simulink library "motion"  (Simulink 4.00)
undefined symbols (not defined in the file or in its folder): A6, Ac, Acd, ad, Aff, Aff0, Aff6, Ap, As, B6, Bc, Bcd, Bff, Bff0, Bff6, Bp, Bs, C6, Cc, Ccd, Cff, Cff0, Cff6, Cp, Cs, D6, Dc, dd, Ddd, Dff, Dff0, Dff6, Dp, Ds, jd, Ts, Tsettle
libraries: motion x5
(part 3 of 4)

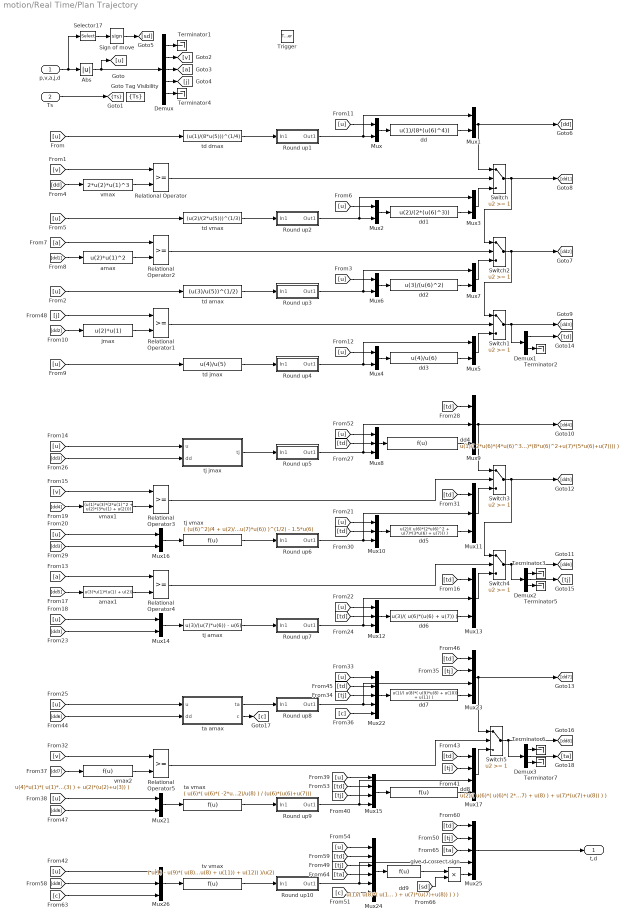
== system motion/Real Time/Plan Trajectory ==
  p,v,a,j,d : Inport  Port=1
  Ts : Inport  Port=2
  Trigger : TriggerPort  TriggerType=rising  OutputDataType=auto
  Abs : Abs  SaturateOnIntegerOverflow=on
  Demux : Demux  Outputs=5  BusSelectionMode=off
  Demux1 : Demux  Outputs=2  BusSelectionMode=off
  Demux2 : Demux  Outputs=3  BusSelectionMode=off
  Demux3 : Demux  Outputs=[2 1 1]  BusSelectionMode=off
  Goto Tag Visibility : GotoTagVisibility  GotoTag=Ts
  Mux{,1..7,14,16,21} (11 alike) : Mux  Inputs=2
  Mux{8..13,26} (7 alike) : Mux  Inputs=3
  Mux15 : Mux  Inputs=4
  Mux17 : Mux  Inputs=4
  Mux22 : Mux  Inputs=5
  Mux23 : Mux  Inputs=4
  Mux24 : Mux  Inputs=6
  Mux25 : Mux  Inputs=5
  Relational Operator{,1..5} (6 alike) : RelationalOperator  Operator=>=
  Round up1 : Subsystem
      settings: RTWFcnNameOpts=Auto  RTWFileNameOpts=Auto
      mask Display: disp('Ts*ceil(u/Ts)')
  Round up10 : Subsystem
      settings: RTWFcnNameOpts=Auto  RTWFileNameOpts=Auto
      mask Display: disp('Ts*ceil(u/Ts)')
  Round up2 : Subsystem
      settings: RTWFcnNameOpts=Auto  RTWFileNameOpts=Auto
      mask Display: disp('Ts*ceil(u/Ts)')
  Round up3 : Subsystem
      settings: RTWFcnNameOpts=Auto  RTWFileNameOpts=Auto
      mask Display: disp('Ts*ceil(u/Ts)')
  Round up4 : Subsystem
      settings: RTWFcnNameOpts=Auto  RTWFileNameOpts=Auto
      mask Display: disp('Ts*ceil(u/Ts)')
  Round up5 : Subsystem
      settings: RTWFcnNameOpts=Auto  RTWFileNameOpts=Auto
      mask Display: disp('Ts*ceil(u/Ts)')
  Round up6 : Subsystem
      settings: RTWFcnNameOpts=Auto  RTWFileNameOpts=Auto
      mask Display: disp('Ts*ceil(u/Ts)')
  Round up7 : Subsystem
      settings: RTWFcnNameOpts=Auto  RTWFileNameOpts=Auto
      mask Display: disp('Ts*ceil(u/Ts)')
  Round up8 : Subsystem
      settings: RTWFcnNameOpts=Auto  RTWFileNameOpts=Auto
      mask Display: disp('Ts*ceil(u/Ts)')
  Round up9 : Subsystem
      settings: RTWFcnNameOpts=Auto  RTWFileNameOpts=Auto
      mask Display: disp('Ts*ceil(u/Ts)')
  Selector17 : Selector  InputType=Vector  ElementSrc=Internal  Elements=1  RowSrc=Internal  Rows=1  ColumnSrc=Internal  Columns=1  InputPortWidth=5
  Sign of move : Signum
  Switch{,1..5} (6 alike) : Switch  Threshold=1
  Terminator{1..7} (7 alike) : Terminator
  amax : Fcn  Expr=u(2)*u(1)^2
  amax1 : Fcn  Expr=u(3)*u(1)*(u(1) + u(2))
  dd : Fcn  Expr=u(1)/(8*(u(6)^4))
  dd1 : Fcn  Expr=u(2)/(2*(u(6)^3))
  dd2 : Fcn  Expr=u(3)/(u(6)^2)
  dd3 : Fcn  Expr=u(4)/u(6)
  dd4 : Fcn  Expr=u(1)/( 2*u(6)*(4*u(6)^3+u(7)*(8*u(6)^2+u(7)*(5*u(6)+u(7)))) )
  dd5 : Fcn  Expr=u(2)/( u(6)*(2*u(6)^2 + u(7)*(3*u(6) + u(7))) )
  dd6 : Fcn  Expr=u(3)/( u(6)*(u(6) + u(7)) )
  dd7 : Fcn  Expr=u(1)/( u(8)*( u(9)*u(8) + u(10)) + u(11) )
  dd8 : Fcn  Expr=u(2)/( u(6)*( u(6)*( 2*u(6) + 3*u(7) + u(8) ) + u(7)*(u(7)+u(8)) ) )
  dd9 : Fcn  Expr=u(1)/( u(8)*( u(10)*u(8) + u(11)) + u(12) + u(9)*( u(6)*( u(6)*( 2*u(6) + 3*u(7) + u(8) ) + u(7)*(u(7)+u(8)) ) ) )
  give d correct sign : Product  Inputs=2  Multiplication=Element-wise(.*)  SaturateOnIntegerOverflow=on
  jmax : Fcn  Expr=u(2)*u(1)
  ta amax : Subsystem
      settings: RTWFcnNameOpts=Auto  RTWFileNameOpts=Auto
  ta vmax : Fcn  Expr=( u(6)*( u(6)*( -2*u(6) - 3*u(7) ) - u(7)^2 ) + u(2)/u(8) ) / (u(6)*(u(6)+u(7)))
  td amax : Fcn  Expr=(u(3)/u(5))^(1/2)
  td dmax : Fcn  Expr=(u(1)/(8*u(5)))^(1/4)
  td jmax : Fcn  Expr=u(4)/u(5)
  td vmax : Fcn  Expr=(u(2)/(2*u(5)))^(1/3)
  tj amax : Fcn  Expr=u(3)/(u(7)*u(6)) - u(6)
  tj jmax : Subsystem
      settings: RTWFcnNameOpts=Auto  RTWFileNameOpts=Auto
  tj vmax : Fcn  Expr=( (u(6)^2)/4 + u(2)/(u(7)*u(6)) )^(1/2) - 1.5*u(6)
  tv vmax : Fcn  Expr=( u(1) - u(9)*( u(8)*(u(10)*u(8) + u(11)) + u(12)) )/u(2)
  vmax : Fcn  Expr=2*u(2)*u(1)^3
  vmax1 : Fcn  Expr=(u(1)*u(3)*(2*u(1)^2 + u(2)*(3*u(1) + u(2))))
  vmax2 : Fcn  Expr=u(4)*u(1)*( u(1)*( 2*u(1) + 3*u(2) + u(3) ) + u(2)*(u(2)+u(3)) )
  t,d : Outport  Port=1
  tag scope: Ts=scoped
  wires:
  [sd] -> give d correct sign/2
  dd9/1 -> give d correct sign/1
  give d correct sign/1 -> Mux25/5
  [ta] -> Mux25/3
  [tj] -> Mux25/2
  [td] -> Mux25/1
  Mux25/1 -> t,d/1
  Sign of move/1 -> [sd]
  Selector17/1 -> Sign of move/1
  p,v,a,j,d/1 -> Selector17/1, Abs/1
  Abs/1 -> Demux/1, [u]
  Demux/5 -> Terminator4/1
  Demux/4 -> [j]
  Demux/3 -> [a]
  Demux/2 -> [v]
  Demux/1 -> Terminator1/1
  Ts/1 -> [Ts]
  Round up10/1(Out1) -> Mux24/5, Mux25/4
  tv vmax/1 -> Round up10/1(In1)
  Round up9/1(Out1) -> Mux15/4, Mux17/3
  ta vmax/1 -> Round up9/1(In1)
  Round up8/1(Out1) -> Mux22/4, Mux23/3
  ta amax/1(ta) -> Round up8/1(In1)
  Round up7/1(Out1) -> Mux12/3, Mux13/2
  tj amax/1 -> Round up7/1(In1)
  Round up6/1(Out1) -> Mux10/3, Mux11/2
  tj vmax/1 -> Round up6/1(In1)
  Round up5/1(Out1) -> Mux8/3, Mux9/2
  tj jmax/1(tj) -> Round up5/1(In1)
  Round up4/1(Out1) -> Mux4/2, Mux5/1
  td jmax/1 -> Round up4/1(In1)
  Round up3/1(Out1) -> Mux7/1, Mux6/2
  td amax/1 -> Round up3/1(In1)
  Round up2/1(Out1) -> Mux2/2, Mux3/1
  vmax2/1 -> Relational Operator5/2
  [v] -> Relational Operator5/1
  amax1/1 -> Relational Operator4/2
  [a] -> Relational Operator4/1
  vmax1/1 -> Relational Operator3/2
  [v] -> Relational Operator3/1
  [u] -> Mux24/1
  [u] -> Mux26/1
  Demux3/3 -> Terminator7/1
  Demux3/1 -> Terminator6/1
  Demux3/2 -> [ta]
  Switch5/1 -> Demux3/1, [dd8]
  Relational Operator5/1 -> Switch5/2
  Mux17/1 -> Switch5/3
  [u] -> Mux22/1
  [tj] -> Mux17/2
  [td] -> Mux17/1
  [tj] -> Mux15/3
  ta amax/2(c) -> [c]
  [c] -> Mux22/5
  [tj] -> Mux23/2
  [tj] -> Mux22/3
  [td] -> Mux15/2
  [dd6] -> Mux21/2
  Mux21/1 -> ta vmax/1
  [u] -> Mux21/1
  [td] -> Mux23/1
  [td] -> Mux22/2
  [dd6] -> ta amax/2(dd)
  Mux15/1 -> dd8/1
  dd8/1 -> Mux17/4
  [u] -> Mux15/1
  Mux23/1 -> Switch5/1, [dd7]
  [dd7] -> vmax2/1
  dd7/1 -> Mux23/4
  Mux22/1 -> dd7/1
  [u] -> ta amax/1(u)
  Demux2/3 -> Terminator5/1
  Demux2/1 -> Terminator3/1
  Demux2/2 -> [tj]
  Switch4/1 -> Demux2/1, [dd6]
  Relational Operator4/1 -> Switch4/2
  Mux13/1 -> Switch4/3
  Switch3/1 -> Switch4/1, [dd5]
  Relational Operator3/1 -> Switch3/2
  Mux11/1 -> Switch3/3
  [u] -> Mux8/1
  [td] -> Mux13/1
  [td] -> Mux12/2
  [dd3] -> Mux14/2
  Mux14/1 -> tj amax/1
  [u] -> Mux14/1
  Mux12/1 -> dd6/1
  dd6/1 -> Mux13/3
  [u] -> Mux12/1
  [dd5] -> amax1/1
  [td] -> Mux11/1
  [td] -> Mux10/2
  [dd3] -> Mux16/2
  Mux16/1 -> tj vmax/1
  [u] -> Mux16/1
  [td] -> Mux9/1
  [td] -> Mux8/2
  [dd3] -> tj jmax/2(dd)
  Mux10/1 -> dd5/1
  dd5/1 -> Mux11/3
  [u] -> Mux10/1
  Mux9/1 -> Switch3/1, [dd4]
  [dd4] -> vmax1/1
  dd4/1 -> Mux9/3
  Mux8/1 -> dd4/1
  [u] -> tj jmax/1(u)
  Demux1/2 -> Terminator2/1
  Demux1/1 -> [td]
  [u] -> Mux/1
  jmax/1 -> Relational Operator1/2
  [j] -> Relational Operator1/1
  Switch1/1 -> Demux1/1, [dd3]
  Relational Operator1/1 -> Switch1/2
  Mux5/1 -> Switch1/3
  Mux4/1 -> dd3/1
  dd3/1 -> Mux5/2
  [u] -> Mux4/1
  [u] -> td jmax/1
  [dd2] -> jmax/1
  amax/1 -> Relational Operator2/2
  [a] -> Relational Operator2/1
  Switch2/1 -> Switch1/1, [dd2]
  Relational Operator2/1 -> Switch2/2
  Mux7/1 -> Switch2/3
  Mux6/1 -> dd2/1
  dd2/1 -> Mux7/2
  [u] -> Mux6/1
  [u] -> td amax/1
  [dd1] -> amax/1
  vmax/1 -> Relational Operator/2
  [v] -> Relational Operator/1
  Switch/1 -> Switch2/1, [dd1]
  Relational Operator/1 -> Switch/2
  Mux3/1 -> Switch/3
  td vmax/1 -> Round up2/1(In1)
  Mux2/1 -> dd1/1
  dd1/1 -> Mux3/2
  [u] -> Mux2/1
  [u] -> td vmax/1
  Mux1/1 -> Switch/1, [dd]
  [dd] -> vmax/1
  dd/1 -> Mux1/2
  Mux/1 -> dd/1
  Round up1/1(Out1) -> Mux/2, Mux1/1
  td dmax/1 -> Round up1/1(In1)
  [u] -> td dmax/1
  [ta] -> Mux24/4
  [c] -> Mux24/6
  [c] -> Mux26/3
  Mux26/1 -> tv vmax/1
  [tj] -> Mux24/3
  [td] -> Mux24/2
  [dd8] -> Mux26/2
  Mux24/1 -> dd9/1

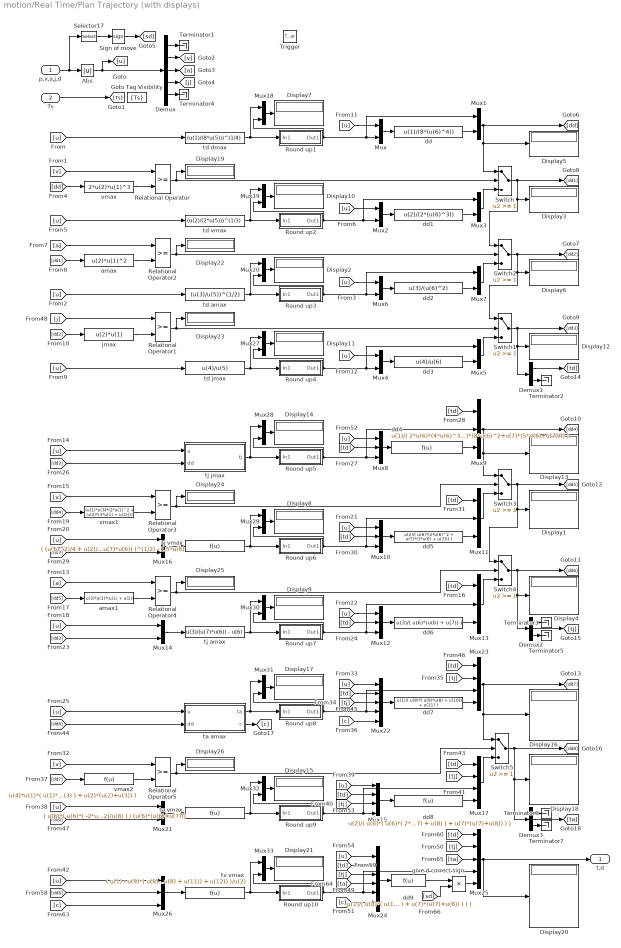
== system motion/Real Time/Plan Trajectory (with displays) ==
  p,v,a,j,d : Inport  Port=1
  Ts : Inport  Port=2
  Trigger : TriggerPort  TriggerType=rising  OutputDataType=auto
  Abs : Abs  SaturateOnIntegerOverflow=on
  Demux : Demux  Outputs=5  BusSelectionMode=off
  Demux1 : Demux  Outputs=2  BusSelectionMode=off
  Demux2 : Demux  Outputs=3  BusSelectionMode=off
  Demux3 : Demux  Outputs=[2 1 1]  BusSelectionMode=off
  Display{1..26} (26 alike) : Display
      settings: Format=short
  Goto Tag Visibility : GotoTagVisibility  GotoTag=Ts
  Mux{,1..7,14,16,18..21,27..33} (21 alike) : Mux  Inputs=2
  Mux{8..13,26} (7 alike) : Mux  Inputs=3
  Mux15 : Mux  Inputs=4
  Mux17 : Mux  Inputs=4
  Mux22 : Mux  Inputs=5
  Mux23 : Mux  Inputs=4
  Mux24 : Mux  Inputs=6
  Mux25 : Mux  Inputs=5
  Relational Operator{,1..5} (6 alike) : RelationalOperator  Operator=>=
  Round up1 : Subsystem
      settings: RTWFcnNameOpts=Auto  RTWFileNameOpts=Auto
      mask Display: disp('Ts*ceil(u/Ts)')
  Round up10 : Subsystem
      settings: RTWFcnNameOpts=Auto  RTWFileNameOpts=Auto
      mask Display: disp('Ts*ceil(u/Ts)')
  Round up2 : Subsystem
      settings: RTWFcnNameOpts=Auto  RTWFileNameOpts=Auto
      mask Display: disp('Ts*ceil(u/Ts)')
  Round up3 : Subsystem
      settings: RTWFcnNameOpts=Auto  RTWFileNameOpts=Auto
      mask Display: disp('Ts*ceil(u/Ts)')
  Round up4 : Subsystem
      settings: RTWFcnNameOpts=Auto  RTWFileNameOpts=Auto
      mask Display: disp('Ts*ceil(u/Ts)')
  Round up5 : Subsystem
      settings: RTWFcnNameOpts=Auto  RTWFileNameOpts=Auto
      mask Display: disp('Ts*ceil(u/Ts)')
  Round up6 : Subsystem
      settings: RTWFcnNameOpts=Auto  RTWFileNameOpts=Auto
      mask Display: disp('Ts*ceil(u/Ts)')
  Round up7 : Subsystem
      settings: RTWFcnNameOpts=Auto  RTWFileNameOpts=Auto
      mask Display: disp('Ts*ceil(u/Ts)')
  Round up8 : Subsystem
      settings: RTWFcnNameOpts=Auto  RTWFileNameOpts=Auto
      mask Display: disp('Ts*ceil(u/Ts)')
  Round up9 : Subsystem
      settings: RTWFcnNameOpts=Auto  RTWFileNameOpts=Auto
      mask Display: disp('Ts*ceil(u/Ts)')
  Selector17 : Selector  InputType=Vector  ElementSrc=Internal  Elements=1  RowSrc=Internal  Rows=1  ColumnSrc=Internal  Columns=1  InputPortWidth=5
  Sign of move : Signum
  Switch{,1..5} (6 alike) : Switch  Threshold=1
  Terminator{1..7} (7 alike) : Terminator
  amax : Fcn  Expr=u(2)*u(1)^2
  amax1 : Fcn  Expr=u(3)*u(1)*(u(1) + u(2))
  dd : Fcn  Expr=u(1)/(8*(u(6)^4))
  dd1 : Fcn  Expr=u(2)/(2*(u(6)^3))
  dd2 : Fcn  Expr=u(3)/(u(6)^2)
  dd3 : Fcn  Expr=u(4)/u(6)
  dd4 : Fcn  Expr=u(1)/( 2*u(6)*(4*u(6)^3+u(7)*(8*u(6)^2+u(7)*(5*u(6)+u(7)))) )
  dd5 : Fcn  Expr=u(2)/( u(6)*(2*u(6)^2 + u(7)*(3*u(6) + u(7))) )
  dd6 : Fcn  Expr=u(3)/( u(6)*(u(6) + u(7)) )
  dd7 : Fcn  Expr=u(1)/( u(8)*( u(9)*u(8) + u(10)) + u(11) )
  dd8 : Fcn  Expr=u(2)/( u(6)*( u(6)*( 2*u(6) + 3*u(7) + u(8) ) + u(7)*(u(7)+u(8)) ) )
  dd9 : Fcn  Expr=u(1)/( u(8)*( u(10)*u(8) + u(11)) + u(12) + u(9)*( u(6)*( u(6)*( 2*u(6) + 3*u(7) + u(8) ) + u(7)*(u(7)+u(8)) ) ) )
  give d correct sign : Product  Inputs=2  Multiplication=Element-wise(.*)  SaturateOnIntegerOverflow=on
  jmax : Fcn  Expr=u(2)*u(1)
  ta amax : Subsystem
      settings: RTWFcnNameOpts=Auto  RTWFileNameOpts=Auto
  ta vmax : Fcn  Expr=( u(6)*( u(6)*( -2*u(6) - 3*u(7) ) - u(7)^2 ) + u(2)/u(8) ) / (u(6)*(u(6)+u(7)))
  td amax : Fcn  Expr=(u(3)/u(5))^(1/2)
  td dmax : Fcn  Expr=(u(1)/(8*u(5)))^(1/4)
  td jmax : Fcn  Expr=u(4)/u(5)
  td vmax : Fcn  Expr=(u(2)/(2*u(5)))^(1/3)
  tj amax : Fcn  Expr=u(3)/(u(7)*u(6)) - u(6)
  tj jmax : Subsystem
      settings: RTWFcnNameOpts=Auto  RTWFileNameOpts=Auto
  tj vmax : Fcn  Expr=( (u(6)^2)/4 + u(2)/(u(7)*u(6)) )^(1/2) - 1.5*u(6)
  tv vmax : Fcn  Expr=( u(1) - u(9)*( u(8)*(u(10)*u(8) + u(11)) + u(12)) )/u(2)
  vmax : Fcn  Expr=2*u(2)*u(1)^3
  vmax1 : Fcn  Expr=(u(1)*u(3)*(2*u(1)^2 + u(2)*(3*u(1) + u(2))))
  vmax2 : Fcn  Expr=u(4)*u(1)*( u(1)*( 2*u(1) + 3*u(2) + u(3) ) + u(2)*(u(2)+u(3)) )
  t,d : Outport  Port=1
  tag scope: Ts=scoped
  wires:
  Mux24/1 -> dd9/1
  [dd8] -> Mux26/2
  [td] -> Mux24/2
  [tj] -> Mux24/3
  Mux26/1 -> tv vmax/1
  [c] -> Mux26/3
  [c] -> Mux24/6
  [ta] -> Mux24/4
  [u] -> td dmax/1
  td dmax/1 -> Mux18/1, Round up1/1(In1)
  Round up1/1(Out1) -> Mux18/2, Mux1/1, Mux/2
  Mux/1 -> dd/1
  dd/1 -> Mux1/2
  [dd] -> vmax/1
  Mux1/1 -> Switch/1, Display5/1, [dd]
  [u] -> td vmax/1
  [u] -> Mux2/1
  dd1/1 -> Mux3/2
  Mux2/1 -> dd1/1
  td vmax/1 -> Round up2/1(In1), Mux19/1
  Mux3/1 -> Switch/3
  Relational Operator/1 -> Display19/1, Switch/2
  Switch/1 -> Switch2/1, Display3/1, [dd1]
  [v] -> Relational Operator/1
  vmax/1 -> Relational Operator/2
  [dd1] -> amax/1
  [u] -> td amax/1
  [u] -> Mux6/1
  dd2/1 -> Mux7/2
  Mux6/1 -> dd2/1
  Mux7/1 -> Switch2/3
  Relational Operator2/1 -> Display22/1, Switch2/2
  Switch2/1 -> Switch1/1, Display6/1, [dd2]
  [a] -> Relational Operator2/1
  amax/1 -> Relational Operator2/2
  [dd2] -> jmax/1
  [u] -> td jmax/1
  [u] -> Mux4/1
  dd3/1 -> Mux5/2
  Mux4/1 -> dd3/1
  Mux5/1 -> Switch1/3
  Relational Operator1/1 -> Display23/1, Switch1/2
  Switch1/1 -> Demux1/1, Display12/1, [dd3]
  [j] -> Relational Operator1/1
  jmax/1 -> Relational Operator1/2
  [u] -> Mux/1
  Demux1/1 -> [td]
  Demux1/2 -> Terminator2/1
  [u] -> tj jmax/1(u)
  Mux8/1 -> dd4/1
  dd4/1 -> Mux9/3
  [dd4] -> vmax1/1
  Mux9/1 -> Switch3/1, Display13/1, [dd4]
  [u] -> Mux10/1
  dd5/1 -> Mux11/3
  Mux10/1 -> dd5/1
  [dd3] -> tj jmax/2(dd)
  [td] -> Mux8/2
  [td] -> Mux9/1
  [u] -> Mux16/1
  Mux16/1 -> tj vmax/1
  [dd3] -> Mux16/2
  [td] -> Mux10/2
  [td] -> Mux11/1
  [dd5] -> amax1/1
  [u] -> Mux12/1
  dd6/1 -> Mux13/3
  Mux12/1 -> dd6/1
  [u] -> Mux14/1
  Mux14/1 -> tj amax/1
  [dd3] -> Mux14/2
  [td] -> Mux12/2
  [td] -> Mux13/1
  [u] -> Mux8/1
  Mux11/1 -> Switch3/3
  Relational Operator3/1 -> Display24/1, Switch3/2
  Switch3/1 -> Switch4/1, Display1/1, [dd5]
  Mux13/1 -> Switch4/3
  Relational Operator4/1 -> Display25/1, Switch4/2
  Switch4/1 -> Demux2/1, Display4/1, [dd6]
  Demux2/2 -> [tj]
  Demux2/1 -> Terminator3/1
  Demux2/3 -> Terminator5/1
  [u] -> ta amax/1(u)
  Mux22/1 -> dd7/1
  dd7/1 -> Mux23/4
  [dd7] -> vmax2/1
  Mux23/1 -> Switch5/1, Display16/1, [dd7]
  [u] -> Mux15/1
  dd8/1 -> Mux17/4
  Mux15/1 -> dd8/1
  [dd6] -> ta amax/2(dd)
  [td] -> Mux22/2
  [td] -> Mux23/1
  [u] -> Mux21/1
  Mux21/1 -> ta vmax/1
  [dd6] -> Mux21/2
  [td] -> Mux15/2
  [tj] -> Mux22/3
  [tj] -> Mux23/2
  [c] -> Mux22/5
  ta amax/2(c) -> [c]
  [tj] -> Mux15/3
  [td] -> Mux17/1
  [tj] -> Mux17/2
  [u] -> Mux22/1
  Mux17/1 -> Switch5/3
  Relational Operator5/1 -> Display26/1, Switch5/2
  Switch5/1 -> Demux3/1, Display18/1, [dd8]
  Demux3/2 -> [ta]
  Demux3/1 -> Terminator6/1
  Demux3/3 -> Terminator7/1
  [u] -> Mux26/1
  [u] -> Mux24/1
  [v] -> Relational Operator3/1
  vmax1/1 -> Relational Operator3/2
  [a] -> Relational Operator4/1
  amax1/1 -> Relational Operator4/2
  [v] -> Relational Operator5/1
  vmax2/1 -> Relational Operator5/2
  Mux18/1 -> Display7/1
  Round up2/1(Out1) -> Mux3/1, Mux2/2, Mux19/2
  Mux19/1 -> Display10/1
  td amax/1 -> Round up3/1(In1), Mux20/1
  Round up3/1(Out1) -> Mux6/2, Mux7/1, Mux20/2
  Mux20/1 -> Display2/1
  td jmax/1 -> Round up4/1(In1), Mux27/1
  Round up4/1(Out1) -> Mux5/1, Mux4/2, Mux27/2
  Mux27/1 -> Display11/1
  tj jmax/1(tj) -> Round up5/1(In1), Mux28/1
  Round up5/1(Out1) -> Mux9/2, Mux8/3, Mux28/2
  Mux28/1 -> Display14/1
  tj vmax/1 -> Round up6/1(In1), Mux29/1
  Round up6/1(Out1) -> Mux11/2, Mux10/3, Mux29/2
  Mux29/1 -> Display8/1
  tj amax/1 -> Round up7/1(In1), Mux30/1
  Round up7/1(Out1) -> Mux13/2, Mux12/3, Mux30/2
  Mux30/1 -> Display9/1
  ta amax/1(ta) -> Round up8/1(In1), Mux31/1
  Round up8/1(Out1) -> Mux23/3, Mux22/4, Mux31/2
  Mux31/1 -> Display17/1
  ta vmax/1 -> Round up9/1(In1), Mux32/1
  Round up9/1(Out1) -> Mux17/3, Mux15/4, Mux32/2
  Mux32/1 -> Display15/1
  tv vmax/1 -> Round up10/1(In1), Mux33/1
  Round up10/1(Out1) -> Mux25/4, Mux24/5, Mux33/2
  Mux33/1 -> Display21/1
  Ts/1 -> [Ts]
  Demux/1 -> Terminator1/1
  Demux/2 -> [v]
  Demux/3 -> [a]
  Demux/4 -> [j]
  Demux/5 -> Terminator4/1
  Abs/1 -> [u], Demux/1
  p,v,a,j,d/1 -> Abs/1, Selector17/1
  Selector17/1 -> Sign of move/1
  Sign of move/1 -> [sd]
  Mux25/1 -> t,d/1, Display20/1
  [td] -> Mux25/1
  [tj] -> Mux25/2
  [ta] -> Mux25/3
  give d correct sign/1 -> Mux25/5
  dd9/1 -> give d correct sign/1
  [sd] -> give d correct sign/2

== system motion/Real Time/X-Y planner  ==
  note: Define waypoints: e.g., t=[1:20]; X=[ sin(t*pi/10)' cos(2*t*pi/10+pi/2)' ];
  "Cont " : Inport  Port=1
  Trig : Inport  Port=2
  Generate Feedforward X : Subsystem  mask{m1=0.10, m2=0.03, k1=1, k2=1, c=2.1e4, k12=0.4, Ts=Ts, S1=1, S2=1}
      mask prompts: m1 "Actuator Mass [kg]"; m2 "Load Mass [kg]"; k1 "Actuator Damping [Ns/m]"; k2 "Load Damping [Ns/m]"; c "Stiffness [N/m]"; k12 "Internal Damping [Ns/m]"; Ts "Sample Time [s]"; S1 "Select: 4th order(1) or rigid body(0)"; S2 "Select: actuator(1) or load(0) pos mmnt"
      settings: RTWFcnNameOpts=Auto  RTWFileNameOpts=Auto
  Generate Feedforward Y : Subsystem  mask{m1=0.22, m2=0.03, k1=1, k2=1, c=1.2e4, k12=1.5, Ts=Ts, S1=1, S2=1}
      mask prompts: m1 "Actuator Mass [kg]"; m2 "Load Mass [kg]"; k1 "Actuator Damping [Ns/m]"; k2 "Load Damping [Ns/m]"; c "Stiffness [N/m]"; k12 "Internal Damping [Ns/m]"; Ts "Sample Time [s]"; S1 "Select: 4th order(1) or rigid body(0)"; S2 "Select: actuator(1) or load(0) pos mmnt"
      settings: RTWFcnNameOpts=Auto  RTWFileNameOpts=Auto
  Generate Profile with reset : motion/Real Time/Generate Profile with reset  Ts=Ts  Tset=Tsettle  Sdir=0
  Memory1 : Memory  X0=0  InheritSampleTime=off
  Mux1 : Mux  Inputs=5
  "Plan Trajectory " : motion/Real Time/Plan Trajectory (with displays)  TreatAsAtomicUnit=on  SimViewingDevice=off
      settings: Permissions=ReadWrite  RTWFcnNameOpts=Auto  RTWFileNameOpts=Auto
  Product2 : Product  Inputs=2  Multiplication=Element-wise(.*)  SaturateOnIntegerOverflow=on
  Product3 : Product  Inputs=2  Multiplication=Element-wise(.*)  SaturateOnIntegerOverflow=on
  Start position : Constant  Value=[0 0]
  Switch1 : Switch  Threshold=.5
  Terminator : Terminator
  Ts : Constant  Value=Ts
  Waypoints : Subsystem  TreatAsAtomicUnit=on  mask{P=X, pmin=0.001}
      mask prompts: P "Waypoints [ [x1 y1] ; [x2 y2] ; .....]"; pmin "Minimal stepsize (>0)"
      mask init:
      | Pm=max(max(abs(P)));
      | X.time=[];
      | X.signals.values=[P/Pm*0.25];
      settings: RTWFcnNameOpts=Auto  RTWFileNameOpts=Auto
  a : Constant  Value=2
  d : Constant  Value=100000
  j : Constant  Value=200
  "single move " : Subsystem
      settings: RTWFcnNameOpts=Auto  RTWFileNameOpts=Auto
  v : Constant  Value=0.2
  X : Outport  Port=1
  Y : Outport  Port=2
  wires:
  [p] -> Mux1/1
  [Y] -> Product3/1
  [X] -> Product2/1
  [start] -> "single move "/2(start)
  Switch1/1 -> Generate Profile with reset/2
  [start] -> Waypoints/Trigger
  "Cont "/1 -> Switch1/1, Switch1/2  "Continuous"
  Trig/1 -> "single move "/1(trigger)  "Single move trigger"
  "single move "/1(enable) -> Switch1/3
  Waypoints/4(pos) -> Terminator/1
  Waypoints/3(Y) -> [Y]
  Waypoints/2(X) -> [X]
  Waypoints/1(p) -> [p]
  Start position/1 -> Waypoints/1(start position)
  Generate Feedforward Y/1(Out) -> Y/1
  Product3/1 -> Generate Feedforward Y/1(djerk)
  Generate Profile with reset/1 -> Product3/2, Product2/2
  Product2/1 -> Generate Feedforward X/1(djerk)
  Generate Feedforward X/1(Out) -> X/1
  Generate Profile with reset/2 -> Generate Feedforward Y/2(reset), Generate Feedforward X/2(reset)
  Generate Profile with reset/3 -> [start]
  Memory1/1 -> Generate Profile with reset/1
  [start] -> "Plan Trajectory "/Trigger
  Mux1/1 -> "Plan Trajectory "/1
  "Plan Trajectory "/1 -> Memory1/1
  d/1 -> Mux1/5
  j/1 -> Mux1/4
  a/1 -> Mux1/3
  Ts/1 -> "Plan Trajectory "/2
  v/1 -> Mux1/2

== system motion/Real Time/open example ==
  note: Run makeplant

== system motion/Real Time/open example1 ==
  note: Run makeplant

== system motion/Feedforward Controllers/2nd order continuous/rigid body ==

== system motion/Feedforward Controllers/2nd order discrete/Discrete variable delay ==
  In1 : Inport  Port=1
  1-alpha : Gain  Gain=1-alpha  Multiplication=Element-wise(K.*u)  SaturateOnIntegerOverflow=on
  Sum1 : Sum  Inputs=++|  SaturateOnIntegerOverflow=on
  Sum2 : Sum  Inputs=+-|  SaturateOnIntegerOverflow=on
  Unit Delay : UnitDelay  X0=0  SampleTime=Ts
  Out1 : Outport  Port=1
  wires:
  In1/1 -> Sum2/1, Unit Delay/1
  Unit Delay/1 -> Sum1/2, Sum2/2
  Sum1/1 -> Out1/1
  1-alpha/1 -> Sum1/1
  Sum2/1 -> 1-alpha/1

== system motion/Feedforward Controllers/2nd order discrete/Discrete variable delay1 ==
  In1 : Inport  Port=1
  1-alpha : Gain  Gain=1-alpha  Multiplication=Element-wise(K.*u)  SaturateOnIntegerOverflow=on
  Sum1 : Sum  Inputs=++|  SaturateOnIntegerOverflow=on
  Sum2 : Sum  Inputs=+-|  SaturateOnIntegerOverflow=on
  Unit Delay : UnitDelay  X0=0  SampleTime=Ts
  Out1 : Outport  Port=1
  wires:
  Sum2/1 -> 1-alpha/1
  1-alpha/1 -> Sum1/1
  Sum1/1 -> Out1/1
  Unit Delay/1 -> Sum2/2, Sum1/2
  In1/1 -> Unit Delay/1, Sum2/1

== system motion/Feedforward Controllers/2nd order discrete/Discrete variable delay2 ==
  In1 : Inport  Port=1
  1-alpha : Gain  Gain=1-alpha  Multiplication=Element-wise(K.*u)  SaturateOnIntegerOverflow=on
  Sum1 : Sum  Inputs=++|  SaturateOnIntegerOverflow=on
  Sum2 : Sum  Inputs=+-|  SaturateOnIntegerOverflow=on
  Unit Delay : UnitDelay  X0=0  SampleTime=Ts
  Out1 : Outport  Port=1
  wires:
  In1/1 -> Sum2/1, Unit Delay/1
  Unit Delay/1 -> Sum1/2, Sum2/2
  Sum1/1 -> Out1/1
  1-alpha/1 -> Sum1/1
  Sum2/1 -> 1-alpha/1

== system motion/Feedforward Controllers/3d order continuous/rigid body ==

== system motion/Feedforward Controllers/3d order discrete/Discrete variable delay ==
  In1 : Inport  Port=1
  1-alpha : Gain  Gain=1-alpha  Multiplication=Element-wise(K.*u)  SaturateOnIntegerOverflow=on
  Sum1 : Sum  Inputs=++|  SaturateOnIntegerOverflow=on
  Sum2 : Sum  Inputs=+-|  SaturateOnIntegerOverflow=on
  Unit Delay : UnitDelay  X0=0  SampleTime=Ts
  Out1 : Outport  Port=1
  wires:
  Sum2/1 -> 1-alpha/1
  1-alpha/1 -> Sum1/1
  Sum1/1 -> Out1/1
  Unit Delay/1 -> Sum2/2, Sum1/2
  In1/1 -> Unit Delay/1, Sum2/1

== system motion/Feedforward Controllers/3d order discrete/Discrete variable delay1 ==
  In1 : Inport  Port=1
  1-alpha : Gain  Gain=1-alpha  Multiplication=Element-wise(K.*u)  SaturateOnIntegerOverflow=on
  Sum1 : Sum  Inputs=++|  SaturateOnIntegerOverflow=on
  Sum2 : Sum  Inputs=+-|  SaturateOnIntegerOverflow=on
  Unit Delay : UnitDelay  X0=0  SampleTime=Ts
  Out1 : Outport  Port=1
  wires:
  In1/1 -> Sum2/1, Unit Delay/1
  Unit Delay/1 -> Sum1/2, Sum2/2
  Sum1/1 -> Out1/1
  1-alpha/1 -> Sum1/1
  Sum2/1 -> 1-alpha/1

== system motion/Feedforward Controllers/3d order discrete/Discrete variable delay2 ==
  In1 : Inport  Port=1
  1-alpha : Gain  Gain=1-alpha  Multiplication=Element-wise(K.*u)  SaturateOnIntegerOverflow=on
  Sum1 : Sum  Inputs=++|  SaturateOnIntegerOverflow=on
  Sum2 : Sum  Inputs=+-|  SaturateOnIntegerOverflow=on
  Unit Delay : UnitDelay  X0=0  SampleTime=Ts
  Out1 : Outport  Port=1
  wires:
  Sum2/1 -> 1-alpha/1
  1-alpha/1 -> Sum1/1
  Sum1/1 -> Out1/1
  Unit Delay/1 -> Sum2/2, Sum1/2
  In1/1 -> Unit Delay/1, Sum2/1

== system motion/Feedforward Controllers/4th order  continuous x1/rigid body ==

== system motion/Feedforward Controllers/4th order  discrete x1/Discrete variable delay ==
  In1 : Inport  Port=1
  1-alpha : Gain  Gain=1-alpha  Multiplication=Element-wise(K.*u)  SaturateOnIntegerOverflow=on
  Sum1 : Sum  Inputs=++|  SaturateOnIntegerOverflow=on
  Sum2 : Sum  Inputs=+-|  SaturateOnIntegerOverflow=on
  Unit Delay : UnitDelay  X0=0  SampleTime=Ts
  Out1 : Outport  Port=1
  wires:
  Sum2/1 -> 1-alpha/1
  1-alpha/1 -> Sum1/1
  Sum1/1 -> Out1/1
  Unit Delay/1 -> Sum2/2, Sum1/2
  In1/1 -> Unit Delay/1, Sum2/1

== system motion/Feedforward Controllers/4th order  discrete x1/Discrete variable delay1 ==
  In1 : Inport  Port=1
  1-alpha : Gain  Gain=1-alpha  Multiplication=Element-wise(K.*u)  SaturateOnIntegerOverflow=on
  Sum1 : Sum  Inputs=++|  SaturateOnIntegerOverflow=on
  Sum2 : Sum  Inputs=+-|  SaturateOnIntegerOverflow=on
  Unit Delay : UnitDelay  X0=0  SampleTime=Ts
  Out1 : Outport  Port=1
  wires:
  In1/1 -> Sum2/1, Unit Delay/1
  Unit Delay/1 -> Sum1/2, Sum2/2
  Sum1/1 -> Out1/1
  1-alpha/1 -> Sum1/1
  Sum2/1 -> 1-alpha/1

== system motion/Feedforward Controllers/4th order  discrete x1/Discrete variable delay2 ==
  In1 : Inport  Port=1
  1-alpha : Gain  Gain=1-alpha  Multiplication=Element-wise(K.*u)  SaturateOnIntegerOverflow=on
  Sum1 : Sum  Inputs=++|  SaturateOnIntegerOverflow=on
  Sum2 : Sum  Inputs=+-|  SaturateOnIntegerOverflow=on
  Unit Delay : UnitDelay  X0=0  SampleTime=Ts
  Out1 : Outport  Port=1
  wires:
  Sum2/1 -> 1-alpha/1
  1-alpha/1 -> Sum1/1
  Sum1/1 -> Out1/1
  Unit Delay/1 -> Sum2/2, Sum1/2
  In1/1 -> Unit Delay/1, Sum2/1

== system motion/Feedforward Controllers/4th order continuous/rigid body ==

== system motion/Feedforward Controllers/4th order digital/Discrete variable delay ==
  In1 : Inport  Port=1
  1-alpha : Gain  Gain=1-alpha  Multiplication=Element-wise(K.*u)  SaturateOnIntegerOverflow=on
  Sum1 : Sum  Inputs=++|  SaturateOnIntegerOverflow=on
  Sum2 : Sum  Inputs=+-|  SaturateOnIntegerOverflow=on
  Unit Delay : UnitDelay  X0=0  SampleTime=Ts
  Out1 : Outport  Port=1
  wires:
  Sum2/1 -> 1-alpha/1
  1-alpha/1 -> Sum1/1
  Sum1/1 -> Out1/1
  Unit Delay/1 -> Sum2/2, Sum1/2
  In1/1 -> Unit Delay/1, Sum2/1

== system motion/Feedforward Controllers/4th order digital/Discrete variable delay1 ==
  In1 : Inport  Port=1
  1-alpha : Gain  Gain=1-alpha  Multiplication=Element-wise(K.*u)  SaturateOnIntegerOverflow=on
  Sum1 : Sum  Inputs=++|  SaturateOnIntegerOverflow=on
  Sum2 : Sum  Inputs=+-|  SaturateOnIntegerOverflow=on
  Unit Delay : UnitDelay  X0=0  SampleTime=Ts
  Out1 : Outport  Port=1
  wires:
  In1/1 -> Sum2/1, Unit Delay/1
  Unit Delay/1 -> Sum1/2, Sum2/2
  Sum1/1 -> Out1/1
  1-alpha/1 -> Sum1/1
  Sum2/1 -> 1-alpha/1

== system motion/Feedforward Controllers/4th order digital/Discrete variable delay2 ==
  In1 : Inport  Port=1
  1-alpha : Gain  Gain=1-alpha  Multiplication=Element-wise(K.*u)  SaturateOnIntegerOverflow=on
  Sum1 : Sum  Inputs=++|  SaturateOnIntegerOverflow=on
  Sum2 : Sum  Inputs=+-|  SaturateOnIntegerOverflow=on
  Unit Delay : UnitDelay  X0=0  SampleTime=Ts
  Out1 : Outport  Port=1
  wires:
  Sum2/1 -> 1-alpha/1
  1-alpha/1 -> Sum1/1
  Sum1/1 -> Out1/1
  Unit Delay/1 -> Sum2/2, Sum1/2
  In1/1 -> Unit Delay/1, Sum2/1

== system motion/Feedforward Controllers/4th order discrete/Discrete variable delay ==
  In1 : Inport  Port=1
  1-alpha : Gain  Gain=1-alpha  Multiplication=Element-wise(K.*u)  SaturateOnIntegerOverflow=on
  Sum1 : Sum  Inputs=++|  SaturateOnIntegerOverflow=on
  Sum2 : Sum  Inputs=+-|  SaturateOnIntegerOverflow=on
  Unit Delay : UnitDelay  X0=0  SampleTime=Ts
  Out1 : Outport  Port=1
  wires:
  In1/1 -> Sum2/1, Unit Delay/1
  Unit Delay/1 -> Sum1/2, Sum2/2
  Sum1/1 -> Out1/1
  1-alpha/1 -> Sum1/1
  Sum2/1 -> 1-alpha/1

== system motion/Feedforward Controllers/4th order discrete/Discrete variable delay1 ==
  In1 : Inport  Port=1
  1-alpha : Gain  Gain=1-alpha  Multiplication=Element-wise(K.*u)  SaturateOnIntegerOverflow=on
  Sum1 : Sum  Inputs=++|  SaturateOnIntegerOverflow=on
  Sum2 : Sum  Inputs=+-|  SaturateOnIntegerOverflow=on
  Unit Delay : UnitDelay  X0=0  SampleTime=Ts
  Out1 : Outport  Port=1
  wires:
  Sum2/1 -> 1-alpha/1
  1-alpha/1 -> Sum1/1
  Sum1/1 -> Out1/1
  Unit Delay/1 -> Sum2/2, Sum1/2
  In1/1 -> Unit Delay/1, Sum2/1

== system motion/Feedforward Controllers/4th order discrete/Discrete variable delay2 ==
  In1 : Inport  Port=1
  1-alpha : Gain  Gain=1-alpha  Multiplication=Element-wise(K.*u)  SaturateOnIntegerOverflow=on
  Sum1 : Sum  Inputs=++|  SaturateOnIntegerOverflow=on
  Sum2 : Sum  Inputs=+-|  SaturateOnIntegerOverflow=on
  Unit Delay : UnitDelay  X0=0  SampleTime=Ts
  Out1 : Outport  Port=1
  wires:
  In1/1 -> Sum2/1, Unit Delay/1
  Unit Delay/1 -> Sum1/2, Sum2/2
  Sum1/1 -> Out1/1
  1-alpha/1 -> Sum1/1
  Sum2/1 -> 1-alpha/1

== system motion/General/4th order Digital Feedforward/Discrete variable delay ==
  In1 : Inport  Port=1
  1-alpha : Gain  Gain=1-alpha  Multiplication=Element-wise(K.*u)  SaturateOnIntegerOverflow=on
  Sum1 : Sum  Inputs=++|  SaturateOnIntegerOverflow=on
  Sum2 : Sum  Inputs=+-|  SaturateOnIntegerOverflow=on
  Unit Delay : UnitDelay  X0=0  SampleTime=Ts
  Out1 : Outport  Port=1
  wires:
  Sum2/1 -> 1-alpha/1
  1-alpha/1 -> Sum1/1
  Sum1/1 -> Out1/1
  Unit Delay/1 -> Sum2/2, Sum1/2
  In1/1 -> Unit Delay/1, Sum2/1

== system motion/General/4th order Digital Feedforward/Discrete variable delay1 ==
  In1 : Inport  Port=1
  1-alpha : Gain  Gain=1-alpha  Multiplication=Element-wise(K.*u)  SaturateOnIntegerOverflow=on
  Sum1 : Sum  Inputs=++|  SaturateOnIntegerOverflow=on
  Sum2 : Sum  Inputs=+-|  SaturateOnIntegerOverflow=on
  Unit Delay : UnitDelay  X0=0  SampleTime=Ts
  Out1 : Outport  Port=1
  wires:
  In1/1 -> Sum2/1, Unit Delay/1
  Unit Delay/1 -> Sum1/2, Sum2/2
  Sum1/1 -> Out1/1
  1-alpha/1 -> Sum1/1
  Sum2/1 -> 1-alpha/1

== system motion/General/4th order Digital Feedforward/Discrete variable delay2 ==
  In1 : Inport  Port=1
  1-alpha : Gain  Gain=1-alpha  Multiplication=Element-wise(K.*u)  SaturateOnIntegerOverflow=on
  Sum1 : Sum  Inputs=++|  SaturateOnIntegerOverflow=on
  Sum2 : Sum  Inputs=+-|  SaturateOnIntegerOverflow=on
  Unit Delay : UnitDelay  X0=0  SampleTime=Ts
  Out1 : Outport  Port=1
  wires:
  Sum2/1 -> 1-alpha/1
  1-alpha/1 -> Sum1/1
  Sum1/1 -> Out1/1
  Unit Delay/1 -> Sum2/2, Sum1/2
  In1/1 -> Unit Delay/1, Sum2/1

== system motion/General/4th order Digital Feedforward/Profile Generator ==
  dJerk with error correction : motion/Profile Generators/dJerk with error correction  t0=t0  x=x  v=v  a=a  j=j  d=d  Ts=Ts  r=r  s=s
  profile : Outport  Port=1
  wires:
  dJerk with error correction/1 -> profile/1

== system motion/Real Time/Generate Feedforward/Discrete variable delay1 ==
  In1 : Inport  Port=1
  1-alpha : Gain  Gain=1-alpha  Multiplication=Element-wise(K.*u)  SaturateOnIntegerOverflow=on
  Sum1 : Sum  Inputs=++|  SaturateOnIntegerOverflow=on
  Sum2 : Sum  Inputs=+-|  SaturateOnIntegerOverflow=on
  Unit Delay : UnitDelay  X0=0  SampleTime=Ts
  Out1 : Outport  Port=1
  wires:
  In1/1 -> Sum2/1, Unit Delay/1
  Unit Delay/1 -> Sum1/2, Sum2/2
  Sum1/1 -> Out1/1
  1-alpha/1 -> Sum1/1
  Sum2/1 -> 1-alpha/1

== system motion/Real Time/Generate Feedforward/Discrete variable delay2 ==
  In1 : Inport  Port=1
  1-alpha : Gain  Gain=1-alpha  Multiplication=Element-wise(K.*u)  SaturateOnIntegerOverflow=on
  Sum1 : Sum  Inputs=++|  SaturateOnIntegerOverflow=on
  Sum2 : Sum  Inputs=+-|  SaturateOnIntegerOverflow=on
  Unit Delay : UnitDelay  X0=0  SampleTime=Ts
  Out1 : Outport  Port=1
  wires:
  Sum2/1 -> 1-alpha/1
  1-alpha/1 -> Sum1/1
  Sum1/1 -> Out1/1
  Unit Delay/1 -> Sum2/2, Sum1/2
  In1/1 -> Unit Delay/1, Sum2/1

== system motion/Real Time/Generate Feedforward/Discrete variable delay4 ==
  In1 : Inport  Port=1
  1-alpha : Gain  Gain=1-alpha  Multiplication=Element-wise(K.*u)  SaturateOnIntegerOverflow=on
  Sum1 : Sum  Inputs=++|  SaturateOnIntegerOverflow=on
  Sum2 : Sum  Inputs=+-|  SaturateOnIntegerOverflow=on
  Unit Delay : UnitDelay  X0=0  SampleTime=Ts
  Out1 : Outport  Port=1
  wires:
  In1/1 -> Sum2/1, Unit Delay/1
  Unit Delay/1 -> Sum1/2, Sum2/2
  Sum1/1 -> Out1/1
  1-alpha/1 -> Sum1/1
  Sum2/1 -> 1-alpha/1

== system motion/Real Time/Generate Feedforward with reset/Discrete variable delay1 ==
  In1 : Inport  Port=1
  1-alpha : Gain  Gain=1-alpha  Multiplication=Element-wise(K.*u)  SaturateOnIntegerOverflow=on
  Sum1 : Sum  Inputs=++|  SaturateOnIntegerOverflow=on
  Sum2 : Sum  Inputs=+-|  SaturateOnIntegerOverflow=on
  Unit Delay : UnitDelay  X0=0  SampleTime=Ts
  Out1 : Outport  Port=1
  wires:
  Sum2/1 -> 1-alpha/1
  1-alpha/1 -> Sum1/1
  Sum1/1 -> Out1/1
  Unit Delay/1 -> Sum2/2, Sum1/2
  In1/1 -> Unit Delay/1, Sum2/1

== system motion/Real Time/Generate Feedforward with reset/Discrete variable delay2 ==
  In1 : Inport  Port=1
  1-alpha : Gain  Gain=1-alpha  Multiplication=Element-wise(K.*u)  SaturateOnIntegerOverflow=on
  Sum1 : Sum  Inputs=++|  SaturateOnIntegerOverflow=on
  Sum2 : Sum  Inputs=+-|  SaturateOnIntegerOverflow=on
  Unit Delay : UnitDelay  X0=0  SampleTime=Ts
  Out1 : Outport  Port=1
  wires:
  In1/1 -> Sum2/1, Unit Delay/1
  Unit Delay/1 -> Sum1/2, Sum2/2
  Sum1/1 -> Out1/1
  1-alpha/1 -> Sum1/1
  Sum2/1 -> 1-alpha/1

== system motion/Real Time/Generate Feedforward with reset/Discrete variable delay4 ==
  In1 : Inport  Port=1
  1-alpha : Gain  Gain=1-alpha  Multiplication=Element-wise(K.*u)  SaturateOnIntegerOverflow=on
  Sum1 : Sum  Inputs=++|  SaturateOnIntegerOverflow=on
  Sum2 : Sum  Inputs=+-|  SaturateOnIntegerOverflow=on
  Unit Delay : UnitDelay  X0=0  SampleTime=Ts
  Out1 : Outport  Port=1
  wires:
  Sum2/1 -> 1-alpha/1
  1-alpha/1 -> Sum1/1
  Sum1/1 -> Out1/1
  Unit Delay/1 -> Sum2/2, Sum1/2
  In1/1 -> Unit Delay/1, Sum2/1

== system motion/Real Time/Generate Feedforward with reset/acceleration ==
  in : Inport  Port=1
  reset : Inport  Port=2
  Constant : Constant  Value=0
  Constant1 : Constant  Value=0
  Gain4 : Gain  Gain=Ts/2  Multiplication=Element-wise(K.*u)  SaturateOnIntegerOverflow=on
  Sum : Sum  Inputs=|++  SaturateOnIntegerOverflow=on
  Sum1 : Sum  Inputs=|-+  SaturateOnIntegerOverflow=on
  Sum6 : Sum  Inputs=+-  SaturateOnIntegerOverflow=on
  Switch : Switch  Threshold=.5
  Switch1 : Switch  Threshold=.5
  Unit Delay4 : UnitDelay  X0=0  SampleTime=Ts
  Unit Delay5 : UnitDelay  X0=0  SampleTime=Ts
  out : Outport  Port=1
  wires:
  Constant/1 -> Switch/1
  Sum/1 -> Switch/3
  reset/1 -> Switch/2, Switch1/2
  Constant1/1 -> Switch1/1
  Sum1/1 -> Switch1/3
  Gain4/1 -> Sum/1, Sum1/1
  in/1 -> Gain4/1
  Sum6/1 -> out/1
  Unit Delay5/1 -> Sum1/2, Sum6/2
  Switch/1 -> Unit Delay4/1
  Switch1/1 -> Unit Delay5/1
  Unit Delay4/1 -> Sum6/1, Sum/2

== system motion/Real Time/Generate Feedforward with reset/jerk ==
  in : Inport  Port=1
  reset : Inport  Port=2
  Constant : Constant  Value=0
  Constant1 : Constant  Value=0
  Gain4 : Gain  Gain=Ts/2  Multiplication=Element-wise(K.*u)  SaturateOnIntegerOverflow=on
  Sum : Sum  Inputs=|++  SaturateOnIntegerOverflow=on
  Sum1 : Sum  Inputs=|-+  SaturateOnIntegerOverflow=on
  Sum6 : Sum  Inputs=+-  SaturateOnIntegerOverflow=on
  Switch : Switch  Threshold=.5
  Switch1 : Switch  Threshold=.5
  Unit Delay4 : UnitDelay  X0=0  SampleTime=Ts
  Unit Delay5 : UnitDelay  X0=0  SampleTime=Ts
  out : Outport  Port=1
  wires:
  Unit Delay4/1 -> Sum/2, Sum6/1
  Switch1/1 -> Unit Delay5/1
  Switch/1 -> Unit Delay4/1
  Unit Delay5/1 -> Sum6/2, Sum1/2
  Sum6/1 -> out/1
  in/1 -> Gain4/1
  Gain4/1 -> Sum1/1, Sum/1
  Sum1/1 -> Switch1/3
  Constant1/1 -> Switch1/1
  reset/1 -> Switch1/2, Switch/2
  Sum/1 -> Switch/3
  Constant/1 -> Switch/1

== system motion/Real Time/Generate Feedforward with reset/position ==
  in : Inport  Port=1
  reset : Inport  Port=2
  Constant : Constant  Value=0
  Constant1 : Constant  Value=0
  Gain4 : Gain  Gain=Ts/2  Multiplication=Element-wise(K.*u)  SaturateOnIntegerOverflow=on
  Sum : Sum  Inputs=|++  SaturateOnIntegerOverflow=on
  Sum1 : Sum  Inputs=|-+  SaturateOnIntegerOverflow=on
  Sum6 : Sum  Inputs=+-  SaturateOnIntegerOverflow=on
  Switch : Switch  Threshold=.5
  Switch1 : Switch  Threshold=.5
  Unit Delay4 : UnitDelay  X0=0  SampleTime=Ts
  Unit Delay5 : UnitDelay  X0=0  SampleTime=Ts
  out : Outport  Port=1
  wires:
  Constant/1 -> Switch/1
  Sum/1 -> Switch/3
  reset/1 -> Switch/2, Switch1/2
  Constant1/1 -> Switch1/1
  Sum1/1 -> Switch1/3
  Gain4/1 -> Sum/1, Sum1/1
  in/1 -> Gain4/1
  Sum6/1 -> out/1
  Unit Delay5/1 -> Sum1/2, Sum6/2
  Switch/1 -> Unit Delay4/1
  Switch1/1 -> Unit Delay5/1
  Unit Delay4/1 -> Sum6/1, Sum/2

== system motion/Real Time/Generate Feedforward with reset/velocity ==
  in : Inport  Port=1
  reset : Inport  Port=2
  Constant : Constant  Value=0
  Constant1 : Constant  Value=0
  Gain4 : Gain  Gain=Ts/2  Multiplication=Element-wise(K.*u)  SaturateOnIntegerOverflow=on
  Sum : Sum  Inputs=|++  SaturateOnIntegerOverflow=on
  Sum1 : Sum  Inputs=|-+  SaturateOnIntegerOverflow=on
  Sum6 : Sum  Inputs=+-  SaturateOnIntegerOverflow=on
  Switch : Switch  Threshold=.5
  Switch1 : Switch  Threshold=.5
  Unit Delay4 : UnitDelay  X0=0  SampleTime=Ts
  Unit Delay5 : UnitDelay  X0=0  SampleTime=Ts
  out : Outport  Port=1
  wires:
  Unit Delay4/1 -> Sum/2, Sum6/1
  Switch1/1 -> Unit Delay5/1
  Switch/1 -> Unit Delay4/1
  Unit Delay5/1 -> Sum6/2, Sum1/2
  Sum6/1 -> out/1
  in/1 -> Gain4/1
  Gain4/1 -> Sum1/1, Sum/1
  Sum1/1 -> Switch1/3
  Constant1/1 -> Switch1/1
  reset/1 -> Switch1/2, Switch/2
  Sum/1 -> Switch/3
  Constant/1 -> Switch/1

== system motion/Real Time/Generate Profile/Determine  direction ==
  Trigger : TriggerPort  TriggerType=rising  OutputDataType=auto
  Constant : Constant  Value=-1
  Constant1 : Constant  Value=1
  Memory : Memory  X0=1  InheritSampleTime=on
  Switch : Switch  Threshold=0
  dir : Outport  Port=1
  wires:
  Switch/1 -> Memory/1
  Constant/1 -> Switch/1
  Constant1/1 -> Switch/3
  Memory/1 -> Switch/2, dir/1

== system motion/Real Time/Generate Profile/Enable start ==
  In : Inport  Port=1
  Enable : EnablePort
  Out : Outport  Port=1  OutputWhenDisabled=reset  InitialOutput=0
  wires:
  In/1 -> Out/1

== system motion/Real Time/Generate Profile/Generate start ==
  In : Inport  Port=1
  Constant19 : Constant  Value=0
  Memory2 : Memory  X0=0  InheritSampleTime=off
  Relational Operator16 : RelationalOperator  Operator=>
  Sum1 : Sum  Inputs=|+-  SaturateOnIntegerOverflow=on
  Out : Outport  Port=1
  wires:
  Relational Operator16/1 -> Out/1
  Constant19/1 -> Relational Operator16/2
  Sum1/1 -> Relational Operator16/1
  In/1 -> Memory2/1, Sum1/1
  Memory2/1 -> Sum1/2

== system motion/Real Time/Generate Profile/hold values 1 ==
  In1 : Inport  Port=1
  Trigger : TriggerPort  TriggerType=rising  OutputDataType=auto
  Out1 : Outport  Port=1
  wires:
  In1/1 -> Out1/1

== system motion/Real Time/Generate Profile/hold values 2 ==
  In1 : Inport  Port=1
  Trigger : TriggerPort  TriggerType=rising  OutputDataType=auto
  Out1 : Outport  Port=1
  wires:
  In1/1 -> Out1/1

== system motion/Real Time/Generate Profile with reset/Determine  direction ==
  Trigger : TriggerPort  TriggerType=rising  OutputDataType=auto
  Constant : Constant  Value=-1
  Constant1 : Constant  Value=1
  Memory : Memory  X0=1  InheritSampleTime=on
  Switch : Switch  Threshold=0
  dir : Outport  Port=1
  wires:
  Memory/1 -> dir/1, Switch/2
  Constant1/1 -> Switch/3
  Constant/1 -> Switch/1
  Switch/1 -> Memory/1

== system motion/Real Time/Generate Profile with reset/Enable start ==
  In : Inport  Port=1
  Enable : EnablePort
  Out : Outport  Port=1  OutputWhenDisabled=reset  InitialOutput=0
  wires:
  In/1 -> Out/1

== system motion/Real Time/Generate Profile with reset/Generate start ==
  In : Inport  Port=1
  Constant19 : Constant  Value=0
  Memory2 : Memory  X0=0  InheritSampleTime=off
  Relational Operator16 : RelationalOperator  Operator=>
  Sum1 : Sum  Inputs=|+-  SaturateOnIntegerOverflow=on
  Out : Outport  Port=1
  wires:
  Memory2/1 -> Sum1/2
  In/1 -> Sum1/1, Memory2/1
  Sum1/1 -> Relational Operator16/1
  Constant19/1 -> Relational Operator16/2
  Relational Operator16/1 -> Out/1

== system motion/Real Time/Generate Profile with reset/hold values 1 ==
  In1 : Inport  Port=1
  Trigger : TriggerPort  TriggerType=rising  OutputDataType=auto
  Out1 : Outport  Port=1
  wires:
  In1/1 -> Out1/1

== system motion/Real Time/Generate Profile with reset/hold values 2 ==
  In1 : Inport  Port=1
  Trigger : TriggerPort  TriggerType=rising  OutputDataType=auto
  Out1 : Outport  Port=1
  wires:
  In1/1 -> Out1/1

== system motion/Real Time/Plan Trajectory/Round up1 ==
  In1 : Inport  Port=1
  Product : Product  Inputs=*/  Multiplication=Element-wise(.*)  SaturateOnIntegerOverflow=on
  Product1 : Product  Inputs=**  Multiplication=Element-wise(.*)  SaturateOnIntegerOverflow=on
  Round up : Rounding  Operator=ceil
  Out1 : Outport  Port=1
  wires:
  Product1/1 -> Out1/1
  In1/1 -> Product/1
  Round up/1 -> Product1/1
  Product/1 -> Round up/1
  [Ts] -> Product/2, Product1/2

== system motion/Real Time/Plan Trajectory/Round up10 ==
  In1 : Inport  Port=1
  Product : Product  Inputs=*/  Multiplication=Element-wise(.*)  SaturateOnIntegerOverflow=on
  Product1 : Product  Inputs=**  Multiplication=Element-wise(.*)  SaturateOnIntegerOverflow=on
  Round up : Rounding  Operator=ceil
  Out1 : Outport  Port=1
  wires:
  [Ts] -> Product1/2, Product/2
  Product/1 -> Round up/1
  Round up/1 -> Product1/1
  In1/1 -> Product/1
  Product1/1 -> Out1/1

== system motion/Real Time/Plan Trajectory/Round up2 ==
  In1 : Inport  Port=1
  Product : Product  Inputs=*/  Multiplication=Element-wise(.*)  SaturateOnIntegerOverflow=on
  Product1 : Product  Inputs=**  Multiplication=Element-wise(.*)  SaturateOnIntegerOverflow=on
  Round up : Rounding  Operator=ceil
  Out1 : Outport  Port=1
  wires:
  [Ts] -> Product1/2, Product/2
  Product/1 -> Round up/1
  Round up/1 -> Product1/1
  In1/1 -> Product/1
  Product1/1 -> Out1/1

== system motion/Real Time/Plan Trajectory/Round up3 ==
  In1 : Inport  Port=1
  Product : Product  Inputs=*/  Multiplication=Element-wise(.*)  SaturateOnIntegerOverflow=on
  Product1 : Product  Inputs=**  Multiplication=Element-wise(.*)  SaturateOnIntegerOverflow=on
  Round up : Rounding  Operator=ceil
  Out1 : Outport  Port=1
  wires:
  Product1/1 -> Out1/1
  In1/1 -> Product/1
  Round up/1 -> Product1/1
  Product/1 -> Round up/1
  [Ts] -> Product/2, Product1/2

== system motion/Real Time/Plan Trajectory/Round up4 ==
  In1 : Inport  Port=1
  Product : Product  Inputs=*/  Multiplication=Element-wise(.*)  SaturateOnIntegerOverflow=on
  Product1 : Product  Inputs=**  Multiplication=Element-wise(.*)  SaturateOnIntegerOverflow=on
  Round up : Rounding  Operator=ceil
  Out1 : Outport  Port=1
  wires:
  [Ts] -> Product1/2, Product/2
  Product/1 -> Round up/1
  Round up/1 -> Product1/1
  In1/1 -> Product/1
  Product1/1 -> Out1/1

== system motion/Real Time/Plan Trajectory/Round up5 ==
  In1 : Inport  Port=1
  Product : Product  Inputs=*/  Multiplication=Element-wise(.*)  SaturateOnIntegerOverflow=on
  Product1 : Product  Inputs=**  Multiplication=Element-wise(.*)  SaturateOnIntegerOverflow=on
  Round up : Rounding  Operator=ceil
  Out1 : Outport  Port=1
  wires:
  Product1/1 -> Out1/1
  In1/1 -> Product/1
  Round up/1 -> Product1/1
  Product/1 -> Round up/1
  [Ts] -> Product/2, Product1/2

== system motion/Real Time/Plan Trajectory/Round up6 ==
  In1 : Inport  Port=1
  Product : Product  Inputs=*/  Multiplication=Element-wise(.*)  SaturateOnIntegerOverflow=on
  Product1 : Product  Inputs=**  Multiplication=Element-wise(.*)  SaturateOnIntegerOverflow=on
  Round up : Rounding  Operator=ceil
  Out1 : Outport  Port=1
  wires:
  [Ts] -> Product1/2, Product/2
  Product/1 -> Round up/1
  Round up/1 -> Product1/1
  In1/1 -> Product/1
  Product1/1 -> Out1/1

== system motion/Real Time/Plan Trajectory/Round up7 ==
  In1 : Inport  Port=1
  Product : Product  Inputs=*/  Multiplication=Element-wise(.*)  SaturateOnIntegerOverflow=on
  Product1 : Product  Inputs=**  Multiplication=Element-wise(.*)  SaturateOnIntegerOverflow=on
  Round up : Rounding  Operator=ceil
  Out1 : Outport  Port=1
  wires:
  Product1/1 -> Out1/1
  In1/1 -> Product/1
  Round up/1 -> Product1/1
  Product/1 -> Round up/1
  [Ts] -> Product/2, Product1/2

== system motion/Real Time/Plan Trajectory/Round up8 ==
  In1 : Inport  Port=1
  Product : Product  Inputs=*/  Multiplication=Element-wise(.*)  SaturateOnIntegerOverflow=on
  Product1 : Product  Inputs=**  Multiplication=Element-wise(.*)  SaturateOnIntegerOverflow=on
  Round up : Rounding  Operator=ceil
  Out1 : Outport  Port=1
  wires:
  [Ts] -> Product1/2, Product/2
  Product/1 -> Round up/1
  Round up/1 -> Product1/1
  In1/1 -> Product/1
  Product1/1 -> Out1/1

== system motion/Real Time/Plan Trajectory/Round up9 ==
  In1 : Inport  Port=1
  Product : Product  Inputs=*/  Multiplication=Element-wise(.*)  SaturateOnIntegerOverflow=on
  Product1 : Product  Inputs=**  Multiplication=Element-wise(.*)  SaturateOnIntegerOverflow=on
  Round up : Rounding  Operator=ceil
  Out1 : Outport  Port=1
  wires:
  Product1/1 -> Out1/1
  In1/1 -> Product/1
  Round up/1 -> Product1/1
  Product/1 -> Round up/1
  [Ts] -> Product/2, Product1/2

== system motion/Real Time/Plan Trajectory/ta amax ==
  u : Inport  Port=1
  dd : Inport  Port=2
  Mux1 : Mux  Inputs=3
  Mux17 : Mux  Inputs=3
  c1 : Fcn  Expr=u(1)*(u(1)+u(2))
  c2 : Fcn  Expr=3*u(1)*( 2*u(1)^2 + u(2)*(3*u(1) + u(2)) )
  c3 : Fcn  Expr=2*u(1)*( u(1)*( 4*u(1)^2 + u(2)*(8*u(1) + 5*u(2)) ) + u(2)^3 )
  ta calc : Fcn  Expr=(-u(10) + sqrt(u(10)^2-4*u(9)*(u(11)-u(1)/u(8))))/(2*u(9))
  ta : Outport  Port=1
  c : Outport  Port=2
  wires:
  u/1 -> [u]
  dd/1 -> [dd]
  [dd] -> c1/1, c2/1, c3/1
  Mux1/1 -> ta calc/1
  [u] -> Mux1/1
  [c] -> Mux1/3
  ta calc/1 -> ta/1
  c2/1 -> Mux17/2
  c3/1 -> Mux17/3
  c1/1 -> Mux17/1
  Mux17/1 -> [c], c/1
  [dd] -> Mux1/2

== system motion/Real Time/Plan Trajectory/tj jmax ==
  u : Inport  Port=1
  dd : Inport  Port=2
  D : Fcn  Expr=sqrt(u(1)^3+u(2)^2)
  Demux : Demux  Outputs=5  BusSelectionMode=off
  Demux1 : Demux  Outputs=2  BusSelectionMode=off
  Mux1 : Mux  Inputs=2
  Mux12 : Mux  Inputs=2
  Mux2 : Mux  Inputs=2
  Mux3 : Mux  Inputs=3
  P : Fcn  Expr=-1/9*u(1)^2
  Q : Fcn  Expr=-1/27*u(1)^3-u(3)/(4*u(2)*u(1))
  R : Fcn  Expr=(-u(1)+u(2))^(1/3)
  Terminator{,1..4} (5 alike) : Terminator
  tj calc : Fcn  Expr=u(2) - u(1)/u(2) - 5/3*u(3)
  tj : Outport  Port=1
  wires:
  u/1 -> Demux/1
  Demux/1 -> [p]
  Demux/2 -> Terminator2/1  "v"
  Demux/3 -> Terminator1/1  "a"
  Demux/4 -> Terminator/1  "j"
  Demux/5 -> Terminator3/1  "d"
  dd/1 -> Demux1/1, [dd]
  Demux1/2 -> Terminator4/1  "dd"
  Demux1/1 -> [td]
  [dd] -> P/1, Mux12/1
  Mux12/1 -> Q/1
  [p] -> Mux12/2
  P/1 -> [P]
  Q/1 -> [Q]
  Mux1/1 -> D/1
  [P] -> Mux1/1
  [Q] -> Mux1/2
  D/1 -> [D]
  Mux2/1 -> R/1
  [Q] -> Mux2/1
  [D] -> Mux2/2
  R/1 -> [R]
  Mux3/1 -> tj calc/1
  [P] -> Mux3/1
  [R] -> Mux3/2
  tj calc/1 -> tj/1
  [td] -> Mux3/3

== system motion/Real Time/Plan Trajectory (with displays)/Round up1 ==
  In1 : Inport  Port=1
  Product : Product  Inputs=*/  Multiplication=Element-wise(.*)  SaturateOnIntegerOverflow=on
  Product1 : Product  Inputs=**  Multiplication=Element-wise(.*)  SaturateOnIntegerOverflow=on
  Round up : Rounding  Operator=ceil
  Out1 : Outport  Port=1
  wires:
  [Ts] -> Product1/2, Product/2
  Product/1 -> Round up/1
  Round up/1 -> Product1/1
  In1/1 -> Product/1
  Product1/1 -> Out1/1

== system motion/Real Time/Plan Trajectory (with displays)/Round up10 ==
  In1 : Inport  Port=1
  Product : Product  Inputs=*/  Multiplication=Element-wise(.*)  SaturateOnIntegerOverflow=on
  Product1 : Product  Inputs=**  Multiplication=Element-wise(.*)  SaturateOnIntegerOverflow=on
  Round up : Rounding  Operator=ceil
  Out1 : Outport  Port=1
  wires:
  Product1/1 -> Out1/1
  In1/1 -> Product/1
  Round up/1 -> Product1/1
  Product/1 -> Round up/1
  [Ts] -> Product/2, Product1/2

== system motion/Real Time/Plan Trajectory (with displays)/Round up2 ==
  In1 : Inport  Port=1
  Product : Product  Inputs=*/  Multiplication=Element-wise(.*)  SaturateOnIntegerOverflow=on
  Product1 : Product  Inputs=**  Multiplication=Element-wise(.*)  SaturateOnIntegerOverflow=on
  Round up : Rounding  Operator=ceil
  Out1 : Outport  Port=1
  wires:
  Product1/1 -> Out1/1
  In1/1 -> Product/1
  Round up/1 -> Product1/1
  Product/1 -> Round up/1
  [Ts] -> Product/2, Product1/2

== system motion/Real Time/Plan Trajectory (with displays)/Round up3 ==
  In1 : Inport  Port=1
  Product : Product  Inputs=*/  Multiplication=Element-wise(.*)  SaturateOnIntegerOverflow=on
  Product1 : Product  Inputs=**  Multiplication=Element-wise(.*)  SaturateOnIntegerOverflow=on
  Round up : Rounding  Operator=ceil
  Out1 : Outport  Port=1
  wires:
  [Ts] -> Product1/2, Product/2
  Product/1 -> Round up/1
  Round up/1 -> Product1/1
  In1/1 -> Product/1
  Product1/1 -> Out1/1

== system motion/Real Time/Plan Trajectory (with displays)/Round up4 ==
  In1 : Inport  Port=1
  Product : Product  Inputs=*/  Multiplication=Element-wise(.*)  SaturateOnIntegerOverflow=on
  Product1 : Product  Inputs=**  Multiplication=Element-wise(.*)  SaturateOnIntegerOverflow=on
  Round up : Rounding  Operator=ceil
  Out1 : Outport  Port=1
  wires:
  Product1/1 -> Out1/1
  In1/1 -> Product/1
  Round up/1 -> Product1/1
  Product/1 -> Round up/1
  [Ts] -> Product/2, Product1/2

== system motion/Real Time/Plan Trajectory (with displays)/Round up5 ==
  In1 : Inport  Port=1
  Product : Product  Inputs=*/  Multiplication=Element-wise(.*)  SaturateOnIntegerOverflow=on
  Product1 : Product  Inputs=**  Multiplication=Element-wise(.*)  SaturateOnIntegerOverflow=on
  Round up : Rounding  Operator=ceil
  Out1 : Outport  Port=1
  wires:
  [Ts] -> Product1/2, Product/2
  Product/1 -> Round up/1
  Round up/1 -> Product1/1
  In1/1 -> Product/1
  Product1/1 -> Out1/1

== system motion/Real Time/Plan Trajectory (with displays)/Round up6 ==
  In1 : Inport  Port=1
  Product : Product  Inputs=*/  Multiplication=Element-wise(.*)  SaturateOnIntegerOverflow=on
  Product1 : Product  Inputs=**  Multiplication=Element-wise(.*)  SaturateOnIntegerOverflow=on
  Round up : Rounding  Operator=ceil
  Out1 : Outport  Port=1
  wires:
  Product1/1 -> Out1/1
  In1/1 -> Product/1
  Round up/1 -> Product1/1
  Product/1 -> Round up/1
  [Ts] -> Product/2, Product1/2
